simulink model "GFLIB_ControllerPIpAW_BAM_FLT"  (Simulink 8.3)
settings: Solver=ode45  StartTime=0.0  StopTime=10.0  RelTol=1e-3
undefined symbols (not defined in the file): fltIntegGain, fltPropGain
settings Model: Creator=B17364  LastModifiedBy=B17364
settings DataIOCC: SignalLoggingSaveFormat=Dataset
settings DebuggingCC: UnderspecifiedInitializationDetection=Simplified  StateNameClashWarn=none
settings GRTTargetCC: CombineOutputUpdateFcns=on  GRTInterface=off

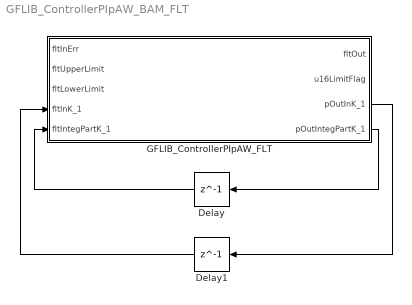
== system GFLIB_ControllerPIpAW_BAM_FLT ==
  Delay : Delay  DelayLength=1  InitialCondition=0
  Delay1 : Delay  DelayLength=1  InitialCondition=0
  GFLIB_ControllerPIpAW_FLT : Subsystem  mask(GFLIB_ControllerPIpAW_FLT){fltPropGain=fltPropGain, fltIntegGain=fltIntegGain}
      mask help: Bit accurate model of parallel form PI controller with anti-windup. All parameters as well as input and output are single precison floating point numbers with exception of u16LimitFlag, which is 16-bit unsigned integer.
      mask init:
      | pos = get_param(gcb, 'Position');width = pos(3) - pos(1); height = pos(4) - pos(2);tX=width/2;tY=height*0.9;
      mask Display: color('black');port_label('input',1,'fltInErr');port_label('input',2,'fltUpperLimit');port_label('input',3,'fltLowerLimit');port_label('input',4,'fltInK_1');port_label('input',5,'fltIntegPartK_1');port_label('output',1,'fltOut');port_label('output',2,'u16LimitFlag');port_label('output',3,'pOutInK_1');port_label('output',4,'pOutIntegPartK_1');color('black');disp('GFLIB_ControllerPIpAW_FLT');color('blue');text(tX,tY, 'BAM', 'horizontalAlignment', 'center');
  wires:
  GFLIB_ControllerPIpAW_FLT/4(pOutIntegPartK_1) -> Delay/1
  GFLIB_ControllerPIpAW_FLT/3(pOutInK_1) -> Delay1/1
  Delay/1 -> GFLIB_ControllerPIpAW_FLT/5(fltIntegPartK_1)
  Delay1/1 -> GFLIB_ControllerPIpAW_FLT/4(fltInK_1)

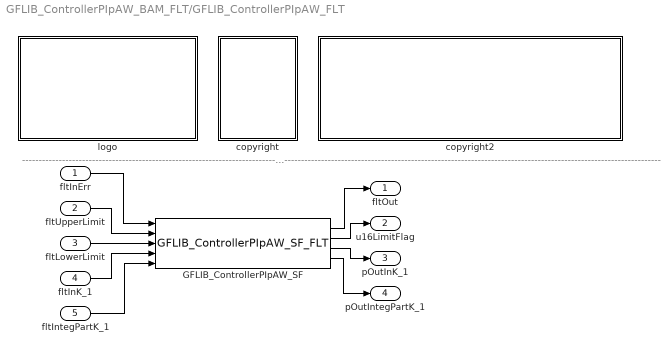
== system GFLIB_ControllerPIpAW_BAM_FLT/GFLIB_ControllerPIpAW_FLT ==
  note: ---------------------------------------------------------------------------------------------------------------------------------------------------------------------------------------------------
  fltInErr : Inport
  fltUpperLimit : Inport  Port=2
  fltLowerLimit : Inport  Port=3
  fltInK_1 : Inport  Port=4
  fltIntegPartK_1 : Inport  Port=5
  GFLIB_ControllerPIpAW_SF : S-Function  FunctionName=GFLIB_ControllerPIpAW_SF_FLT  Parameters=fltPropGain,fltIntegGain  EnableBusSupport=off
  copyright : Subsystem
      mask Display: text(10,90,'FILE:');text(10,75,'DESRIPTION:');text(10,60,'COPYRIGHT:');text(10,45,'VERSION:');text(10,30,'DATE:')
  copyright2 : Subsystem
      mask Display: text(10,90,'GFLIB_ControllerPIpAW_BAM_FLT.mdl');text(10,75,'Parallel form of a standard PI controller with implemented anti-windup.');text(10,60,'Freescale');text(10,45,'0.1');text(10,30,'12-Jun-2015');
  logo : Subsystem
      mask Display: image(imread('logo.jpg'))
  fltOut : Outport
  u16LimitFlag : Outport  Port=2
  pOutInK_1 : Outport  Port=3
  pOutIntegPartK_1 : Outport  Port=4
  wires:
  fltInErr/1 -> GFLIB_ControllerPIpAW_SF/1
  fltUpperLimit/1 -> GFLIB_ControllerPIpAW_SF/2
  fltLowerLimit/1 -> GFLIB_ControllerPIpAW_SF/3
  fltInK_1/1 -> GFLIB_ControllerPIpAW_SF/4
  fltIntegPartK_1/1 -> GFLIB_ControllerPIpAW_SF/5
  GFLIB_ControllerPIpAW_SF/1 -> fltOut/1
  GFLIB_ControllerPIpAW_SF/2 -> u16LimitFlag/1
  GFLIB_ControllerPIpAW_SF/3 -> pOutInK_1/1
  GFLIB_ControllerPIpAW_SF/4 -> pOutIntegPartK_1/1

== system GFLIB_ControllerPIpAW_BAM_FLT/GFLIB_ControllerPIpAW_FLT/copyright ==

== system GFLIB_ControllerPIpAW_BAM_FLT/GFLIB_ControllerPIpAW_FLT/copyright2 ==

== system GFLIB_ControllerPIpAW_BAM_FLT/GFLIB_ControllerPIpAW_FLT/logo ==
